simulink model "Amplitude_Modulation_Simulink"  (R2013a)
settings: Solver=ode45  StartTime=0.0  StopTime=3e-3  MaxStep=0.001e-3  RelTol=1e-3
settings Model: Creator=B407  LastModifiedBy=B407

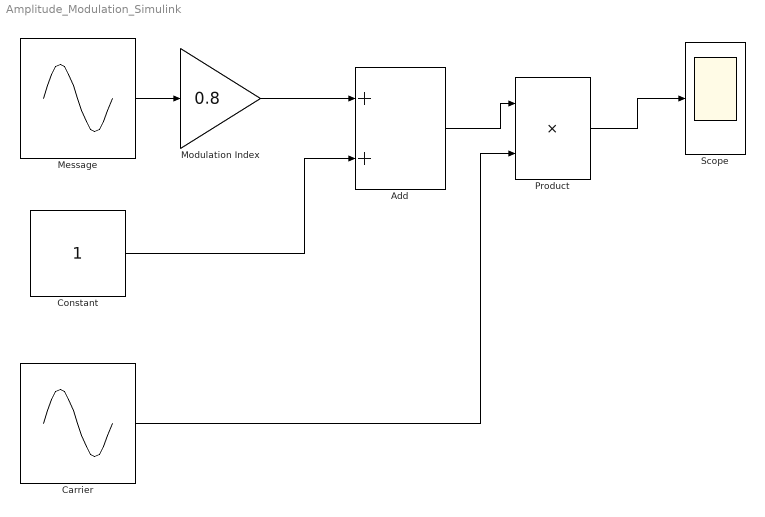
== system Amplitude_Modulation_Simulink ==
  Add : Sum
  "Carrier " : Sin  Frequency=20*6280  Phase=3.14/2  SampleTime=0
  Constant : Constant
  "Message " : Sin  Frequency=6280  Phase=3.14/2  SampleTime=0
  "Modulation Index " : Gain  Gain=0.8
  Product : Product
  Scope : Scope
  wires:
  "Message "/1 -> "Modulation Index "/1
  Constant/1 -> Add/2
  "Modulation Index "/1 -> Add/1
  "Carrier "/1 -> Product/2
  Add/1 -> Product/1
  Product/1 -> Scope/1
